simulink model "Hodgkin_Huxley"  (R2017b)
settings: Solver=VariableStepAuto  StartTime=0.0  StopTime=100  RelTol=1e-3
settings Model: Creator=Lenovo  LastModifiedBy=Lenovo

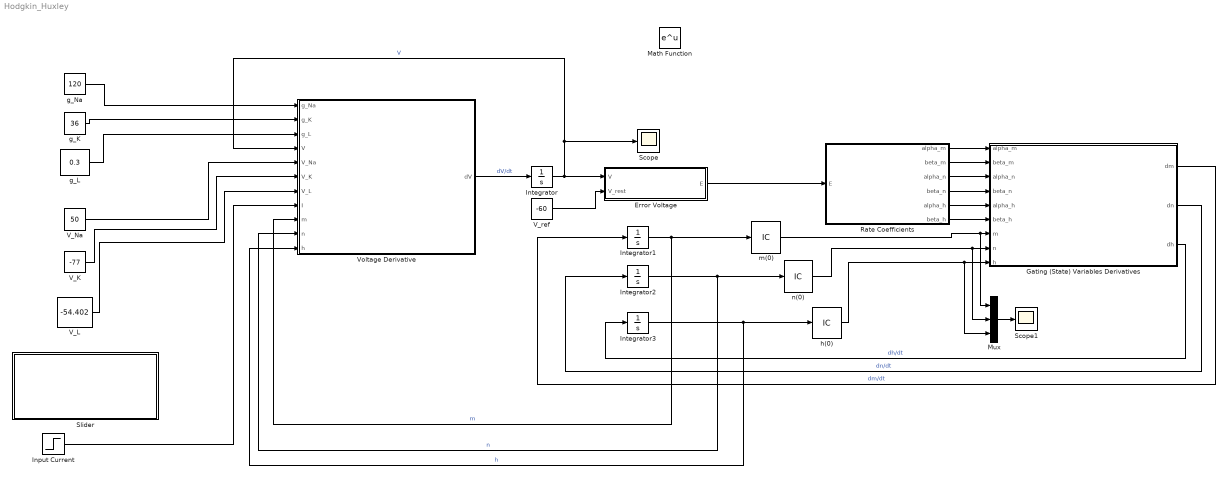
== system Hodgkin_Huxley ==
  Error Voltage : MATLAB Function  TreatAsAtomicUnit=on
  Gating (State) Variables Derivatives : MATLAB Function  TreatAsAtomicUnit=on
  Input Current : Step  Time=50  After=25  SampleTime=0
  Integrator{,1..3} (4 alike) : Integrator
  Math Function : Math  SaturateOnIntegerOverflow=on
  Mux : Mux  Inputs=3
  Rate Coefficients : MATLAB Function  TreatAsAtomicUnit=on
  Scope : Scope
  Scope1 : Scope
  Slider : Subsystem  DialogController=hmiCreateDDGDialog  IsWebBlock=on  mask(MWDashboardBlock){webBlockId=7394cd23-1e0b-4634-aadf-8f0b61d094b3, webBlockType=slider, ShowInLibBrowser=on, ShowInitialText=on, HMISrcModelName=ehe}
      mask prompts: webBlockId "WebBlock Id"; webBlockType "WebBlock Type"; HMISrcModelName "Source Model"
      mask help: SimulinkHMI:dialogs:SliderDialogDesc
      mask Help: helpview([docroot '/mapfiles/simulink.map'], 'hmi_slider')
      mask Display:
      | if strcmp(get_param(bdroot(gcb),'BlockDiagramType'), 'library')
      |     image([(matlabroot) '/toolbox/simulink/hmi/icons/Slider.png']);
      | end
  "V_K " : Constant  Value=-77
  "V_L " : Constant  Value=-54.402
  V_Na : Constant  Value=50
  V_ref : Constant  Value=-60
  "Voltage Derivative " : MATLAB Function  TreatAsAtomicUnit=on
  g_K : Constant  Value=36
  "g_L " : Constant  Value=0.3
  "g_Na " : Constant  Value=120
  h(0) : InitialCondition
  m(0) : InitialCondition  Value=0
  n(0) : InitialCondition  Value=0
  wires:
  V_ref/1 -> Error Voltage/2(V_rest)
  Error Voltage/1(E) -> Rate Coefficients/1(E)
  Rate Coefficients/1(alpha_m) -> Gating (State) Variables Derivatives/1(alpha_m)
  Rate Coefficients/2(beta_m) -> Gating (State) Variables Derivatives/2(beta_m)
  Rate Coefficients/3(alpha_n) -> Gating (State) Variables Derivatives/3(alpha_n)
  Rate Coefficients/4(beta_n) -> Gating (State) Variables Derivatives/4(beta_n)
  Rate Coefficients/5(alpha_h) -> Gating (State) Variables Derivatives/5(alpha_h)
  Rate Coefficients/6(beta_h) -> Gating (State) Variables Derivatives/6(beta_h)
  m(0)/1 -> Mux/1, Gating (State) Variables Derivatives/7(m)
  n(0)/1 -> Mux/2, Gating (State) Variables Derivatives/8(n)
  h(0)/1 -> Mux/3, Gating (State) Variables Derivatives/9(h)
  Gating (State) Variables Derivatives/1(dm) -> Integrator1/1  "dm/dt"
  Gating (State) Variables Derivatives/2(dn) -> Integrator2/1  "dn/dt"
  Gating (State) Variables Derivatives/3(dh) -> Integrator3/1  "dh/dt"
  "g_Na "/1 -> "Voltage Derivative "/1(g_Na)
  g_K/1 -> "Voltage Derivative "/2(g_K)
  "g_L "/1 -> "Voltage Derivative "/3(g_L)
  "Voltage Derivative "/1(dV) -> Integrator/1  "dV/dt"
  V_Na/1 -> "Voltage Derivative "/5(V_Na)
  "V_K "/1 -> "Voltage Derivative "/6(V_K)
  "V_L "/1 -> "Voltage Derivative "/7(V_L)
  Integrator1/1 -> "Voltage Derivative "/9(m), m(0)/1  "m"
  Integrator2/1 -> "Voltage Derivative "/10(n), n(0)/1  "n"
  Integrator3/1 -> "Voltage Derivative "/11(h), h(0)/1  "h"
  Mux/1 -> Scope1/1
  Input Current/1 -> "Voltage Derivative "/8(I)
  Integrator/1 -> Scope/1, "Voltage Derivative "/4(V), Error Voltage/1(V)  "V"

== system Hodgkin_Huxley/Slider ==

== matlab function Hodgkin_Huxley/Error Voltage ==
  data: V input; E output; V_rest input
function E = calcEpsilon(V, V_rest)
E = V - V_rest;

== matlab function Hodgkin_Huxley/Rate Coefficients ==
  data: E input; alpha_m output; beta_m output; alpha_n output; beta_n output; alpha_h output; beta_h output
function [alpha_m, beta_m, alpha_n, beta_n, alpha_h, beta_h] = calcCoeffs(E)
alpha_m = (0.1 * (25 - E )) / (exp((25 - E) / 10) - 1);
beta_m = 4 * exp(-E/18);
alpha_n = (0.01 * (10 - E)) / (exp((10 -E) / 10) - 1);
beta_n = 0.125 * exp(-E / 80);
alpha_h = 0.07 * exp(-E / 20);
beta_h = 1 / (1 + exp((30 - E) / 10));

== matlab function Hodgkin_Huxley/Gating (State) Variables Derivatives ==
  data: alpha_m input; dm output; beta_m input; alpha_n input; beta_n input; alpha_h input; beta_h input; m input; n input; h input; dn output; dh output
function [dm, dn, dh] = calcGatingDer(alpha_m, beta_m, alpha_n, beta_n, alpha_h, beta_h, m, n, h)
dm = alpha_m * (1 - m) - beta_m * m;
dn = alpha_n * (1 - n) - beta_n * n;
dh = alpha_h * (1 - h) - beta_h * h;

== matlab function Hodgkin_Huxley/Voltage Derivative  ==
  data: g_Na input; dV output; g_K input; g_L input; V input; V_Na input; V_K input; V_L input; I input; m input; n input; h input
function dV = calcVoltageDer(g_Na, g_K, g_L, V, V_Na, V_K, V_L, I, m, n, h)
dV = I - g_Na * m^3 * h * (V - V_Na) - g_K * n^4 * (V - V_K) - g_L * (V - V_L);
